simulink model "ballsenkrecht"  (R2014b)
settings: Solver=ode45  StartTime=0.0  StopTime=10.0  RelTol=1e-3
settings Model: Creator=sigurd  LastModifiedBy=sigurd

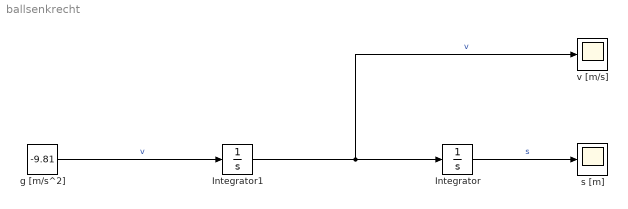
== system ballsenkrecht ==
  Integrator : Integrator  InitialCondition=1.2
  Integrator1 : Integrator  InitialCondition=5
  g [m/s^2] : Constant  Value=-9.81
  s [m] : Scope
  v [m/s] : Scope
  wires:
  Integrator1/1 -> v [m/s]/1, Integrator/1  "v"
  Integrator/1 -> s [m]/1  "s"
  g [m/s^2]/1 -> Integrator1/1  "v"
